simulink model "che381_sim5"  (R2024a)
settings: Solver=VariableStepAuto  StartTime=0.0  StopTime=25  RelTol=1e-3
values from neighbouring files (symbols this model uses):
  Kc = 23    [che381_slab5.m]
  Td = 1.96    [che381_slab5.m]
  Ti = 262    [che381_slab5.m]
settings Model: Creator=Shrimi Agrawal  LastModifiedBy=Shrimi Agrawal

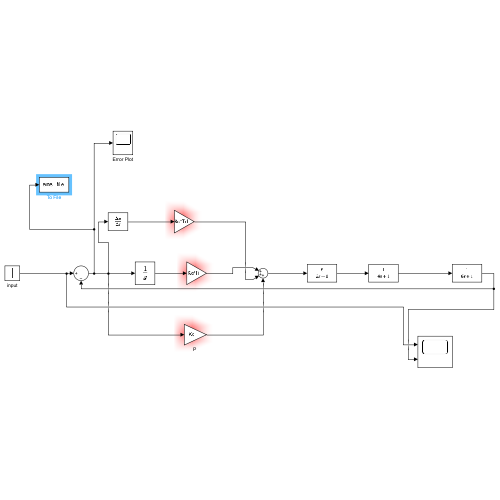
[thumbnail: Simulink's stored preview of the top-level diagram]
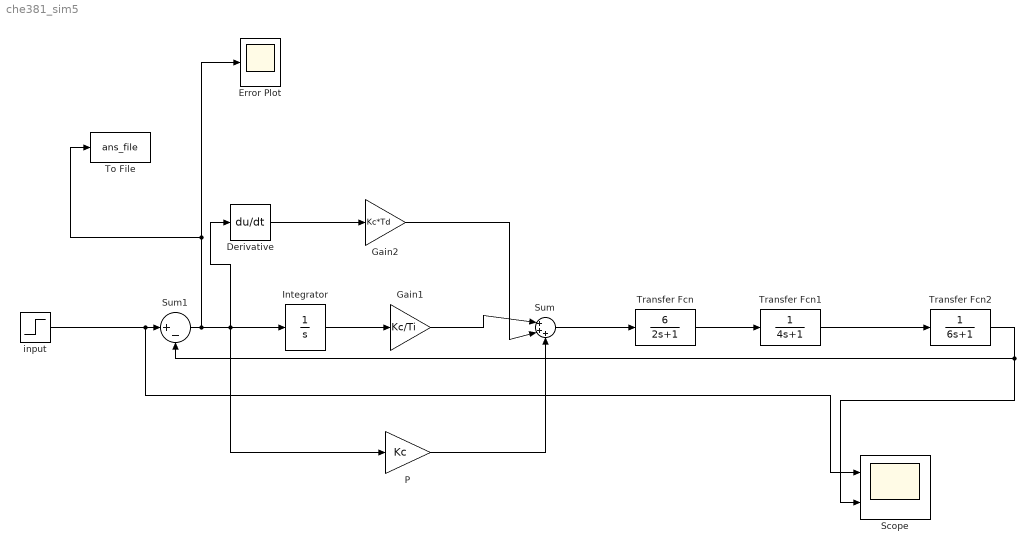
== system che381_sim5 ==
  Derivative : Derivative
  Error Plot : Scope
  Gain1 : Gain  Gain=Kc/Ti
  Gain2 : Gain  Gain=Kc*Td
  Integrator : Integrator
  "P " : Gain  Gain=Kc
  Scope : Scope  NumInputPorts=2
  Sum : Sum  Inputs=|+++
  Sum1 : Sum  Inputs=|+-
  To File : ToFile  Filename=ans_file  SampleTime=0.1
  Transfer Fcn : TransferFcn  Numerator=6  Denominator=[2 1]
  Transfer Fcn1 : TransferFcn  Denominator=[4 1]
  Transfer Fcn2 : TransferFcn  Denominator=[6 1]
  input : Step  SampleTime=0
  wires:
  input/1 -> Scope/1, Sum1/1
  Sum1/1 -> To File/1, Error Plot/1, "P "/1, Derivative/1, Integrator/1
  Integrator/1 -> Gain1/1
  Derivative/1 -> Gain2/1
  Gain1/1 -> Sum/1
  Gain2/1 -> Sum/2
  "P "/1 -> Sum/3
  Sum/1 -> Transfer Fcn/1
  Transfer Fcn/1 -> Transfer Fcn1/1
  Transfer Fcn1/1 -> Transfer Fcn2/1
  Transfer Fcn2/1 -> Scope/2, Sum1/2
